simulink model "tx2"  (R2022a)
settings: Solver=FixedStepDiscrete  StartTime=0.0  StopTime=3.1e6  FixedStep=1  RelTol=1e-3
undefined symbols (not defined in the file or in its folder): rom_bf1, rom_bf2, rom_bf3, rom_bf4, rom_bf5, rom_bf6, rom_bf7, rom_bf8, rom_pilot_tt
libraries: hdlsllib x809, whdlutilities x460, whdlmod x104, whdledac x26, simulink x3
(part 3 of 27)

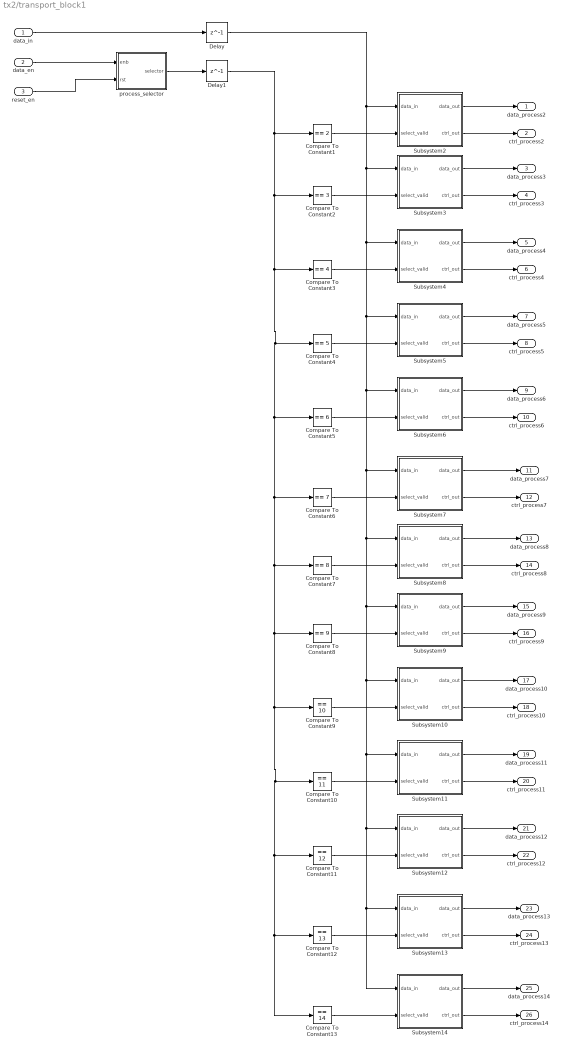
== system tx2/transport_block1 ==
  data_in : Inport  OutDataTypeStr=boolean
  data_en : Inport  Port=2  OutDataTypeStr=boolean
  reset_en : Inport  Port=3  OutDataTypeStr=boolean
  Compare To Constant1 : hdlsllib/Logic and Bit Operations/Compare To Constant  relop===  const=2  OutDataTypeStr=boolean
      settings: SourceProductBaseCode=SL
  Compare To Constant10 : hdlsllib/Logic and Bit Operations/Compare To Constant  relop===  const=11  OutDataTypeStr=boolean
      settings: SourceProductBaseCode=SL
  Compare To Constant11 : hdlsllib/Logic and Bit Operations/Compare To Constant  relop===  const=12  OutDataTypeStr=boolean
      settings: SourceProductBaseCode=SL
  Compare To Constant12 : hdlsllib/Logic and Bit Operations/Compare To Constant  relop===  const=13  OutDataTypeStr=boolean
      settings: SourceProductBaseCode=SL
  Compare To Constant13 : hdlsllib/Logic and Bit Operations/Compare To Constant  relop===  const=14  OutDataTypeStr=boolean
      settings: SourceProductBaseCode=SL
  Compare To Constant2 : hdlsllib/Logic and Bit Operations/Compare To Constant  relop===  const=3  OutDataTypeStr=boolean
      settings: SourceProductBaseCode=SL
  Compare To Constant3 : hdlsllib/Logic and Bit Operations/Compare To Constant  relop===  const=4  OutDataTypeStr=boolean
      settings: SourceProductBaseCode=SL
  Compare To Constant4 : hdlsllib/Logic and Bit Operations/Compare To Constant  relop===  const=5  OutDataTypeStr=boolean
      settings: SourceProductBaseCode=SL
  Compare To Constant5 : hdlsllib/Logic and Bit Operations/Compare To Constant  relop===  const=6  OutDataTypeStr=boolean
      settings: SourceProductBaseCode=SL
  Compare To Constant6 : hdlsllib/Logic and Bit Operations/Compare To Constant  relop===  const=7  OutDataTypeStr=boolean
      settings: SourceProductBaseCode=SL
  Compare To Constant7 : hdlsllib/Logic and Bit Operations/Compare To Constant  relop===  const=8  OutDataTypeStr=boolean
      settings: SourceProductBaseCode=SL
  Compare To Constant8 : hdlsllib/Logic and Bit Operations/Compare To Constant  relop===  const=9  OutDataTypeStr=boolean
      settings: SourceProductBaseCode=SL
  Compare To Constant9 : hdlsllib/Logic and Bit Operations/Compare To Constant  relop===  const=10  OutDataTypeStr=boolean
      settings: SourceProductBaseCode=SL
  Delay : Delay  DelayLength=1  InitialCondition=0
  Delay1 : Delay  DelayLength=1  InitialCondition=0
  Subsystem10 : Subsystem
  Subsystem11 : Subsystem
  Subsystem12 : Subsystem
  Subsystem13 : Subsystem
  Subsystem14 : Subsystem
  Subsystem2 : Subsystem
  Subsystem3 : Subsystem
  Subsystem4 : Subsystem
  Subsystem5 : Subsystem
  Subsystem6 : Subsystem
  Subsystem7 : Subsystem
  Subsystem8 : Subsystem
  Subsystem9 : Subsystem
  process_selector : Subsystem  mask{transblock_len=512, process_len=14}
      mask prompts: transblock_len "the length of the transport block"; process_len "the number of process"
      mask DialogControl ParameterGroupVar Prompt: 参数
  data_process2 : Outport  OutDataTypeStr=boolean  VectorParamsAs1DForOutWhenUnconnected=off
  ctrl_process2 : Outport  Port=2  OutDataTypeStr=Bus: samplecontrol  VectorParamsAs1DForOutWhenUnconnected=off
  data_process3 : Outport  Port=3  OutDataTypeStr=boolean  VectorParamsAs1DForOutWhenUnconnected=off
  ctrl_process3 : Outport  Port=4  OutDataTypeStr=Bus: samplecontrol  VectorParamsAs1DForOutWhenUnconnected=off
  data_process4 : Outport  Port=5  OutDataTypeStr=boolean  VectorParamsAs1DForOutWhenUnconnected=off
  ctrl_process4 : Outport  Port=6  OutDataTypeStr=Bus: samplecontrol  VectorParamsAs1DForOutWhenUnconnected=off
  data_process5 : Outport  Port=7  OutDataTypeStr=boolean  VectorParamsAs1DForOutWhenUnconnected=off
  ctrl_process5 : Outport  Port=8  OutDataTypeStr=Bus: samplecontrol  VectorParamsAs1DForOutWhenUnconnected=off
  data_process6 : Outport  Port=9  OutDataTypeStr=boolean  VectorParamsAs1DForOutWhenUnconnected=off
  ctrl_process6 : Outport  Port=10  OutDataTypeStr=Bus: samplecontrol  VectorParamsAs1DForOutWhenUnconnected=off
  data_process7 : Outport  Port=11  OutDataTypeStr=boolean  VectorParamsAs1DForOutWhenUnconnected=off
  ctrl_process7 : Outport  Port=12  OutDataTypeStr=Bus: samplecontrol  VectorParamsAs1DForOutWhenUnconnected=off
  data_process8 : Outport  Port=13  OutDataTypeStr=boolean  VectorParamsAs1DForOutWhenUnconnected=off
  ctrl_process8 : Outport  Port=14  OutDataTypeStr=Bus: samplecontrol  VectorParamsAs1DForOutWhenUnconnected=off
  data_process9 : Outport  Port=15  OutDataTypeStr=boolean  VectorParamsAs1DForOutWhenUnconnected=off
  ctrl_process9 : Outport  Port=16  OutDataTypeStr=Bus: samplecontrol  VectorParamsAs1DForOutWhenUnconnected=off
  data_process10 : Outport  Port=17  OutDataTypeStr=boolean  VectorParamsAs1DForOutWhenUnconnected=off
  ctrl_process10 : Outport  Port=18  OutDataTypeStr=Bus: samplecontrol  VectorParamsAs1DForOutWhenUnconnected=off
  data_process11 : Outport  Port=19  OutDataTypeStr=boolean  VectorParamsAs1DForOutWhenUnconnected=off
  ctrl_process11 : Outport  Port=20  OutDataTypeStr=Bus: samplecontrol  VectorParamsAs1DForOutWhenUnconnected=off
  data_process12 : Outport  Port=21  OutDataTypeStr=boolean  VectorParamsAs1DForOutWhenUnconnected=off
  ctrl_process12 : Outport  Port=22  OutDataTypeStr=Bus: samplecontrol  VectorParamsAs1DForOutWhenUnconnected=off
  data_process13 : Outport  Port=23  OutDataTypeStr=boolean  VectorParamsAs1DForOutWhenUnconnected=off
  ctrl_process13 : Outport  Port=24  OutDataTypeStr=Bus: samplecontrol  VectorParamsAs1DForOutWhenUnconnected=off
  data_process14 : Outport  Port=25  OutDataTypeStr=boolean  VectorParamsAs1DForOutWhenUnconnected=off
  ctrl_process14 : Outport  Port=26  OutDataTypeStr=Bus: samplecontrol  VectorParamsAs1DForOutWhenUnconnected=off
  wires:
  data_in/1 -> Delay/1
  data_en/1 -> process_selector/1(enb)
  process_selector/1(selector) -> Delay1/1
  Compare To Constant1/1 -> Subsystem2/2(select_valid)
  Subsystem2/1(data_out) -> data_process2/1
  Subsystem2/2(ctrl_out) -> ctrl_process2/1
  Compare To Constant2/1 -> Subsystem3/2(select_valid)
  Subsystem3/1(data_out) -> data_process3/1
  Subsystem3/2(ctrl_out) -> ctrl_process3/1
  Compare To Constant3/1 -> Subsystem4/2(select_valid)
  Subsystem4/1(data_out) -> data_process4/1
  Subsystem4/2(ctrl_out) -> ctrl_process4/1
  Compare To Constant4/1 -> Subsystem5/2(select_valid)
  Subsystem5/1(data_out) -> data_process5/1
  Subsystem5/2(ctrl_out) -> ctrl_process5/1
  Compare To Constant5/1 -> Subsystem6/2(select_valid)
  Subsystem6/1(data_out) -> data_process6/1
  Subsystem6/2(ctrl_out) -> ctrl_process6/1
  Compare To Constant6/1 -> Subsystem7/2(select_valid)
  Subsystem7/1(data_out) -> data_process7/1
  Subsystem7/2(ctrl_out) -> ctrl_process7/1
  Compare To Constant7/1 -> Subsystem8/2(select_valid)
  Subsystem8/1(data_out) -> data_process8/1
  Subsystem8/2(ctrl_out) -> ctrl_process8/1
  Subsystem13/2(ctrl_out) -> ctrl_process13/1
  Subsystem13/1(data_out) -> data_process13/1
  Compare To Constant12/1 -> Subsystem13/2(select_valid)
  Subsystem12/2(ctrl_out) -> ctrl_process12/1
  Subsystem12/1(data_out) -> data_process12/1
  Compare To Constant11/1 -> Subsystem12/2(select_valid)
  Subsystem11/2(ctrl_out) -> ctrl_process11/1
  Subsystem11/1(data_out) -> data_process11/1
  Compare To Constant10/1 -> Subsystem11/2(select_valid)
  Subsystem10/2(ctrl_out) -> ctrl_process10/1
  Subsystem10/1(data_out) -> data_process10/1
  Compare To Constant9/1 -> Subsystem10/2(select_valid)
  Subsystem9/2(ctrl_out) -> ctrl_process9/1
  Subsystem9/1(data_out) -> data_process9/1
  Compare To Constant8/1 -> Subsystem9/2(select_valid)
  reset_en/1 -> process_selector/2(rst)
  Delay1/1 -> Compare To Constant13/1, Compare To Constant12/1, Compare To Constant11/1, Compare To Constant10/1, Compare To Constant9/1, Compare To Constant8/1, Compare To Constant7/1, Compare To Constant6/1, Compare To Constant5/1, Compare To Constant4/1, Compare To Constant3/1, Compare To Constant2/1, Compare To Constant1/1
  Delay/1 -> Subsystem10/1(data_in), Subsystem12/1(data_in), Subsystem14/1(data_in), Subsystem13/1(data_in), Subsystem11/1(data_in), Subsystem9/1(data_in), Subsystem8/1(data_in), Subsystem7/1(data_in), Subsystem6/1(data_in), Subsystem5/1(data_in), Subsystem4/1(data_in), Subsystem3/1(data_in), Subsystem2/1(data_in)
  Compare To Constant13/1 -> Subsystem14/2(select_valid)
  Subsystem14/1(data_out) -> data_process14/1
  Subsystem14/2(ctrl_out) -> ctrl_process14/1

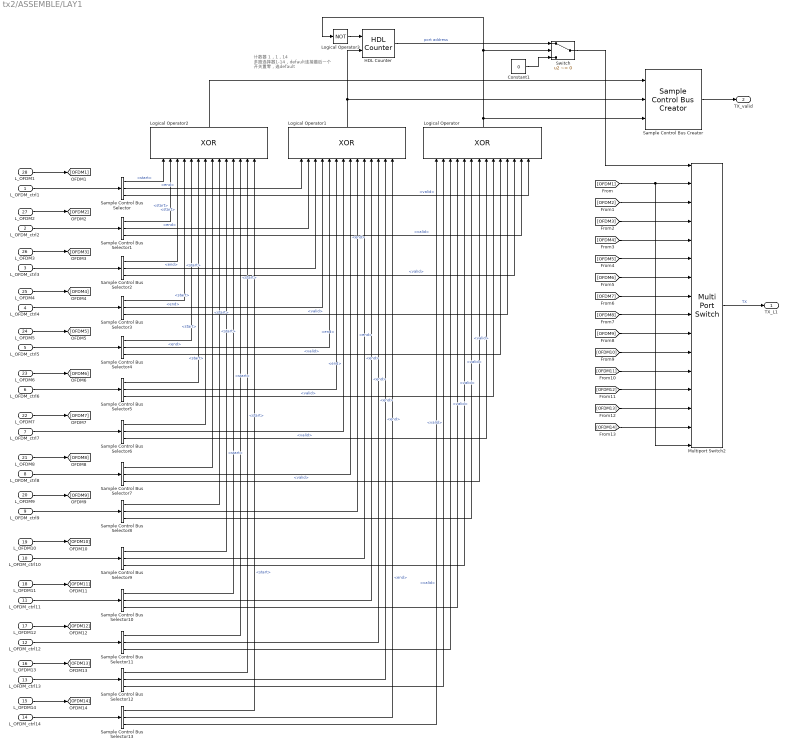
== system tx2/ASSEMBLE/LAY1 ==
  note: 计数器 1，1，14
      | 多路选择器1-14，default连接最后一个
      | 开关置零，选default
  L_OFDM_ctrl1 : Inport  OutDataTypeStr=Bus: samplecontrol
  L_OFDM_ctrl2 : Inport  Port=2  OutDataTypeStr=Bus: samplecontrol
  L_OFDM_ctrl3 : Inport  Port=3  OutDataTypeStr=Bus: samplecontrol
  L_OFDM_ctrl4 : Inport  Port=4  OutDataTypeStr=Bus: samplecontrol
  L_OFDM_ctrl5 : Inport  Port=5  OutDataTypeStr=Bus: samplecontrol
  L_OFDM_ctrl6 : Inport  Port=6  OutDataTypeStr=Bus: samplecontrol
  L_OFDM_ctrl7 : Inport  Port=7  OutDataTypeStr=Bus: samplecontrol
  L_OFDM_ctrl8 : Inport  Port=8  OutDataTypeStr=Bus: samplecontrol
  L_OFDM_ctrl9 : Inport  Port=9  OutDataTypeStr=Bus: samplecontrol
  L_OFDM_ctrl10 : Inport  Port=10  OutDataTypeStr=Bus: samplecontrol
  L_OFDM_ctrl11 : Inport  Port=11  OutDataTypeStr=Bus: samplecontrol
  L_OFDM_ctrl12 : Inport  Port=12  OutDataTypeStr=Bus: samplecontrol
  L_OFDM_ctrl13 : Inport  Port=13  OutDataTypeStr=Bus: samplecontrol
  L_OFDM_ctrl14 : Inport  Port=14  OutDataTypeStr=Bus: samplecontrol
  L_OFDM14 : Inport  Port=15
  L_OFDM13 : Inport  Port=16
  L_OFDM12 : Inport  Port=17
  L_OFDM11 : Inport  Port=18
  L_OFDM10 : Inport  Port=19
  L_OFDM9 : Inport  Port=20
  L_OFDM8 : Inport  Port=21
  L_OFDM7 : Inport  Port=22
  L_OFDM6 : Inport  Port=23
  L_OFDM5 : Inport  Port=24
  L_OFDM4 : Inport  Port=25
  L_OFDM3 : Inport  Port=26
  L_OFDM2 : Inport  Port=27
  L_OFDM1 : Inport  Port=28
  Constant1 : Constant  Value=0  OutDataTypeStr=uint8
  HDL Counter : hdlsllib/Sources/HDL Counter  CountType=Count limited  CountInit=0  CountStep=1  CountMax=13  CountFromType=Initial value  CountFrom=0  CountResetPort=on  CountLoadPort=off  CountEnbPort=on  CountDirPort=off  CountHitOutputPort=off  CountDataType=Unsigned  CountWordLen=8  CountFracLen=0  CountSampTime=1
  Logical Operator : Logic  Operator=XOR  Inputs=14  AllPortsSameDT=off  OutDataTypeStr=boolean
  Logical Operator1 : Logic  Operator=XOR  Inputs=14  AllPortsSameDT=off  OutDataTypeStr=boolean
  Logical Operator2 : Logic  Operator=XOR  Inputs=14  AllPortsSameDT=off  OutDataTypeStr=boolean
  Logical Operator3 : Logic  Operator=NOT  AllPortsSameDT=off  OutDataTypeStr=boolean
  Multiport Switch2 : MultiPortSwitch  DataPortOrder=Zero-based contiguous  Inputs=14  DataPortForDefault=Additional data port  zeroidx=on  SaturateOnIntegerOverflow=off  InputSameDT=off
  Sample Control Bus Creator : whdlutilities/Sample Control Bus Creator
      settings: SourceProductBaseCode=LH
  Sample Control Bus Selector{,1..13} (14 alike) : whdlutilities/Sample Control Bus Selector  OutputSignals=start,end,valid
      settings: SourceProductBaseCode=LH
  Switch : Switch  Criteria=u2 ~= 0  SaturateOnIntegerOverflow=off  InputSameDT=off
  TX_L1 : Outport
  TX_valid : Outport  Port=2  OutDataTypeStr=Bus: samplecontrol
  wires:
  Sample Control Bus Selector8/3 -> Logical Operator/6  "<valid>"
  L_OFDM_ctrl8/1 -> Sample Control Bus Selector7/1
  Sample Control Bus Selector10/3 -> Logical Operator/4  "<valid>"
  L_OFDM5/1 -> [OFDM5]
  Sample Control Bus Selector/3 -> Logical Operator/14  "<valid>"
  Sample Control Bus Selector10/2 -> Logical Operator1/11  "<end>"
  L_OFDM8/1 -> [OFDM8]
  Sample Control Bus Selector1/3 -> Logical Operator/13  "<valid>"
  L_OFDM3/1 -> [OFDM3]
  Sample Control Bus Selector12/3 -> Logical Operator/2  "<valid>"
  L_OFDM2/1 -> [OFDM2]
  Sample Control Bus Selector5/2 -> Logical Operator1/6  "<end>"
  Sample Control Bus Selector6/3 -> Logical Operator/8  "<valid>"
  Logical Operator/1 -> Logical Operator3/1, Switch/2, Sample Control Bus Creator/3
  Sample Control Bus Selector6/2 -> Logical Operator1/7  "<end>"
  L_OFDM10/1 -> [OFDM10]
  Sample Control Bus Selector13/2 -> Logical Operator1/14  "<end>"
  Sample Control Bus Selector12/2 -> Logical Operator1/13  "<end>"
  L_OFDM_ctrl6/1 -> Sample Control Bus Selector5/1
  L_OFDM_ctrl10/1 -> Sample Control Bus Selector9/1
  Sample Control Bus Selector7/3 -> Logical Operator/7  "<valid>"
  Sample Control Bus Selector8/2 -> Logical Operator1/9  "<end>"
  L_OFDM13/1 -> [OFDM13]
  HDL Counter/1 -> Switch/1  "port address"
  Sample Control Bus Selector2/3 -> Logical Operator/12  "<valid>"
  Switch/1 -> Multiport Switch2/1
  Sample Control Bus Selector5/3 -> Logical Operator/9  "<valid>"
  Sample Control Bus Selector/2 -> Logical Operator1/1  "<end>"
  L_OFDM12/1 -> [OFDM12]
  L_OFDM11/1 -> [OFDM11]
  Constant1/1 -> Switch/3
  L_OFDM1/1 -> [OFDM1]
  Sample Control Bus Selector2/2 -> Logical Operator1/3  "<end>"
  Sample Control Bus Selector4/3 -> Logical Operator/10  "<valid>"
  Sample Control Bus Selector11/2 -> Logical Operator1/12  "<end>"
  L_OFDM4/1 -> [OFDM4]
  Sample Control Bus Selector11/3 -> Logical Operator/3  "<valid>"
  Sample Control Bus Selector4/2 -> Logical Operator1/5  "<end>"
  Sample Control Bus Selector3/3 -> Logical Operator/11  "<valid>"
  Sample Control Bus Selector13/3 -> Logical Operator/1  "<valid>"
  Sample Control Bus Selector3/2 -> Logical Operator1/4  "<end>"
  Sample Control Bus Selector1/2 -> Logical Operator1/2  "<end>"
  L_OFDM_ctrl12/1 -> Sample Control Bus Selector11/1
  Sample Control Bus Selector7/2 -> Logical Operator1/8  "<end>"
  L_OFDM_ctrl5/1 -> Sample Control Bus Selector4/1
  Sample Control Bus Selector9/2 -> Logical Operator1/10  "<end>"
  Sample Control Bus Selector9/3 -> Logical Operator/5  "<valid>"
  L_OFDM_ctrl13/1 -> Sample Control Bus Selector12/1
  L_OFDM_ctrl2/1 -> Sample Control Bus Selector1/1
  L_OFDM14/1 -> [OFDM14]
  L_OFDM6/1 -> [OFDM6]
  L_OFDM7/1 -> [OFDM7]
  L_OFDM_ctrl3/1 -> Sample Control Bus Selector2/1
  L_OFDM_ctrl9/1 -> Sample Control Bus Selector8/1
  L_OFDM_ctrl14/1 -> Sample Control Bus Selector13/1
  L_OFDM_ctrl4/1 -> Sample Control Bus Selector3/1
  L_OFDM_ctrl7/1 -> Sample Control Bus Selector6/1
  L_OFDM_ctrl1/1 -> Sample Control Bus Selector/1
  L_OFDM9/1 -> [OFDM9]
  L_OFDM_ctrl11/1 -> Sample Control Bus Selector10/1
  Sample Control Bus Selector/1 -> Logical Operator2/1  "<start>"
  Sample Control Bus Selector1/1 -> Logical Operator2/2  "<start>"
  Sample Control Bus Selector2/1 -> Logical Operator2/3  "<start>"
  Sample Control Bus Selector3/1 -> Logical Operator2/4  "<start>"
  Sample Control Bus Selector4/1 -> Logical Operator2/5  "<start>"
  Sample Control Bus Selector5/1 -> Logical Operator2/6  "<start>"
  Sample Control Bus Selector6/1 -> Logical Operator2/7  "<start>"
  Sample Control Bus Selector7/1 -> Logical Operator2/8  "<start>"
  Sample Control Bus Selector8/1 -> Logical Operator2/9  "<start>"
  Sample Control Bus Selector9/1 -> Logical Operator2/10  "<start>"
  Sample Control Bus Selector10/1 -> Logical Operator2/11  "<start>"
  Sample Control Bus Selector11/1 -> Logical Operator2/12  "<start>"
  Sample Control Bus Selector12/1 -> Logical Operator2/13  "<start>"
  Sample Control Bus Selector13/1 -> Logical Operator2/14  "<start>"
  Sample Control Bus Creator/1 -> TX_valid/1
  Logical Operator2/1 -> Sample Control Bus Creator/1
  [OFDM2] -> Multiport Switch2/3
  [OFDM3] -> Multiport Switch2/4
  Multiport Switch2/1 -> TX_L1/1  "TX"
  Logical Operator3/1 -> HDL Counter/1
  Logical Operator1/1 -> HDL Counter/2, Sample Control Bus Creator/2
  [OFDM4] -> Multiport Switch2/5
  [OFDM5] -> Multiport Switch2/6
  [OFDM6] -> Multiport Switch2/7
  [OFDM7] -> Multiport Switch2/8
  [OFDM8] -> Multiport Switch2/9
  [OFDM9] -> Multiport Switch2/10
  [OFDM10] -> Multiport Switch2/11
  [OFDM11] -> Multiport Switch2/12
  [OFDM12] -> Multiport Switch2/13
  [OFDM13] -> Multiport Switch2/14
  [OFDM14] -> Multiport Switch2/15
  [OFDM1] -> Multiport Switch2/16, Multiport Switch2/2

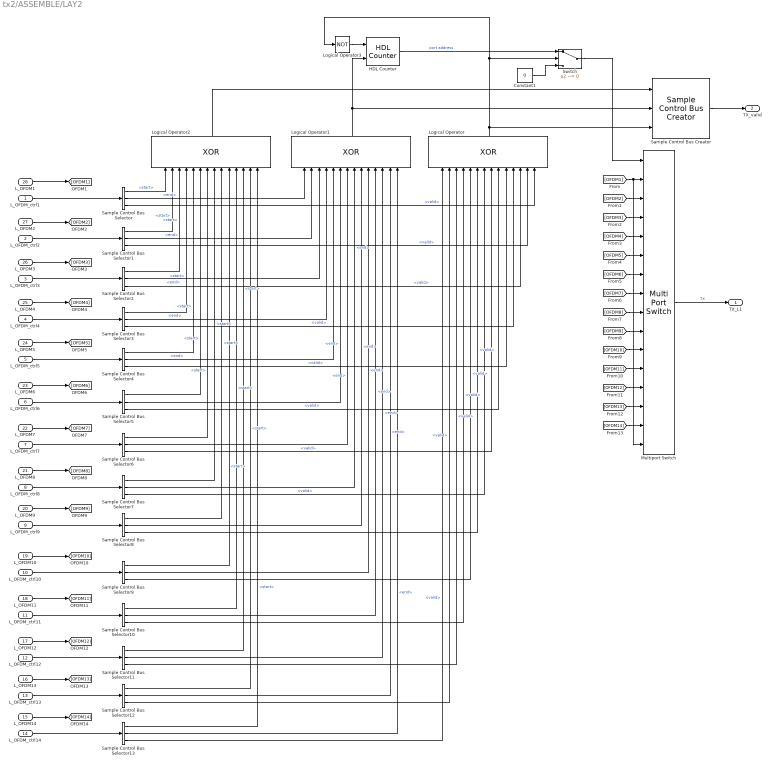
== system tx2/ASSEMBLE/LAY2 ==
  L_OFDM_ctrl1 : Inport  OutDataTypeStr=Bus: samplecontrol
  L_OFDM_ctrl2 : Inport  Port=2  OutDataTypeStr=Bus: samplecontrol
  L_OFDM_ctrl3 : Inport  Port=3  OutDataTypeStr=Bus: samplecontrol
  L_OFDM_ctrl4 : Inport  Port=4  OutDataTypeStr=Bus: samplecontrol
  L_OFDM_ctrl5 : Inport  Port=5  OutDataTypeStr=Bus: samplecontrol
  L_OFDM_ctrl6 : Inport  Port=6  OutDataTypeStr=Bus: samplecontrol
  L_OFDM_ctrl7 : Inport  Port=7  OutDataTypeStr=Bus: samplecontrol
  L_OFDM_ctrl8 : Inport  Port=8  OutDataTypeStr=Bus: samplecontrol
  L_OFDM_ctrl9 : Inport  Port=9  OutDataTypeStr=Bus: samplecontrol
  L_OFDM_ctrl10 : Inport  Port=10  OutDataTypeStr=Bus: samplecontrol
  L_OFDM_ctrl11 : Inport  Port=11  OutDataTypeStr=Bus: samplecontrol
  L_OFDM_ctrl12 : Inport  Port=12  OutDataTypeStr=Bus: samplecontrol
  L_OFDM_ctrl13 : Inport  Port=13  OutDataTypeStr=Bus: samplecontrol
  L_OFDM_ctrl14 : Inport  Port=14  OutDataTypeStr=Bus: samplecontrol
  L_OFDM14 : Inport  Port=15
  L_OFDM13 : Inport  Port=16
  L_OFDM12 : Inport  Port=17
  L_OFDM11 : Inport  Port=18
  L_OFDM10 : Inport  Port=19
  L_OFDM9 : Inport  Port=20
  L_OFDM8 : Inport  Port=21
  L_OFDM7 : Inport  Port=22
  L_OFDM6 : Inport  Port=23
  L_OFDM5 : Inport  Port=24
  L_OFDM4 : Inport  Port=25
  L_OFDM3 : Inport  Port=26
  L_OFDM2 : Inport  Port=27
  L_OFDM1 : Inport  Port=28
  Constant1 : Constant  Value=0  OutDataTypeStr=uint8
  HDL Counter : hdlsllib/Sources/HDL Counter  CountType=Count limited  CountInit=0  CountStep=1  CountMax=13  CountFromType=Initial value  CountFrom=0  CountResetPort=on  CountLoadPort=off  CountEnbPort=on  CountDirPort=off  CountHitOutputPort=off  CountDataType=Unsigned  CountWordLen=8  CountFracLen=0  CountSampTime=1
  Logical Operator : Logic  Operator=XOR  Inputs=14  AllPortsSameDT=off  OutDataTypeStr=boolean
  Logical Operator1 : Logic  Operator=XOR  Inputs=14  AllPortsSameDT=off  OutDataTypeStr=boolean
  Logical Operator2 : Logic  Operator=XOR  Inputs=14  AllPortsSameDT=off  OutDataTypeStr=boolean
  Logical Operator3 : Logic  Operator=NOT  AllPortsSameDT=off  OutDataTypeStr=boolean
  Multiport Switch : MultiPortSwitch  DataPortOrder=Zero-based contiguous  Inputs=14  DataPortForDefault=Additional data port  zeroidx=on  SaturateOnIntegerOverflow=off  InputSameDT=off
  Sample Control Bus Creator : whdlutilities/Sample Control Bus Creator
      settings: SourceProductBaseCode=LH
  Sample Control Bus Selector{,1..13} (14 alike) : whdlutilities/Sample Control Bus Selector  OutputSignals=start,end,valid
      settings: SourceProductBaseCode=LH
  Switch : Switch  Criteria=u2 ~= 0  SaturateOnIntegerOverflow=off  InputSameDT=off
  TX_L1 : Outport
  TX_valid : Outport  Port=2  OutDataTypeStr=Bus: samplecontrol
  wires:
  Logical Operator2/1 -> Sample Control Bus Creator/1
  Sample Control Bus Creator/1 -> TX_valid/1
  Sample Control Bus Selector13/1 -> Logical Operator2/14  "<start>"
  Sample Control Bus Selector12/1 -> Logical Operator2/13  "<start>"
  Sample Control Bus Selector11/1 -> Logical Operator2/12  "<start>"
  Sample Control Bus Selector10/1 -> Logical Operator2/11  "<start>"
  Sample Control Bus Selector9/1 -> Logical Operator2/10  "<start>"
  Sample Control Bus Selector8/1 -> Logical Operator2/9  "<start>"
  Sample Control Bus Selector7/1 -> Logical Operator2/8  "<start>"
  Sample Control Bus Selector6/1 -> Logical Operator2/7  "<start>"
  Sample Control Bus Selector5/1 -> Logical Operator2/6  "<start>"
  Sample Control Bus Selector4/1 -> Logical Operator2/5  "<start>"
  Sample Control Bus Selector3/1 -> Logical Operator2/4  "<start>"
  Sample Control Bus Selector2/1 -> Logical Operator2/3  "<start>"
  Sample Control Bus Selector1/1 -> Logical Operator2/2  "<start>"
  Sample Control Bus Selector/1 -> Logical Operator2/1  "<start>"
  Multiport Switch/1 -> TX_L1/1  "TX"
  L_OFDM_ctrl11/1 -> Sample Control Bus Selector10/1
  L_OFDM9/1 -> [OFDM9]
  L_OFDM_ctrl1/1 -> Sample Control Bus Selector/1
  L_OFDM_ctrl7/1 -> Sample Control Bus Selector6/1
  L_OFDM_ctrl4/1 -> Sample Control Bus Selector3/1
  L_OFDM_ctrl14/1 -> Sample Control Bus Selector13/1
  L_OFDM_ctrl9/1 -> Sample Control Bus Selector8/1
  L_OFDM_ctrl3/1 -> Sample Control Bus Selector2/1
  L_OFDM7/1 -> [OFDM7]
  L_OFDM6/1 -> [OFDM6]
  L_OFDM14/1 -> [OFDM14]
  L_OFDM_ctrl2/1 -> Sample Control Bus Selector1/1
  L_OFDM_ctrl13/1 -> Sample Control Bus Selector12/1
  Sample Control Bus Selector9/3 -> Logical Operator/5  "<valid>"
  Sample Control Bus Selector9/2 -> Logical Operator1/10  "<end>"
  L_OFDM_ctrl5/1 -> Sample Control Bus Selector4/1
  Sample Control Bus Selector7/2 -> Logical Operator1/8  "<end>"
  L_OFDM_ctrl12/1 -> Sample Control Bus Selector11/1
  [OFDM8] -> Multiport Switch/9
  Sample Control Bus Selector1/2 -> Logical Operator1/2  "<end>"
  Sample Control Bus Selector3/2 -> Logical Operator1/4  "<end>"
  Sample Control Bus Selector13/3 -> Logical Operator/1  "<valid>"
  Sample Control Bus Selector3/3 -> Logical Operator/11  "<valid>"
  [OFDM3] -> Multiport Switch/4
  Sample Control Bus Selector4/2 -> Logical Operator1/5  "<end>"
  Sample Control Bus Selector11/3 -> Logical Operator/3  "<valid>"
  [OFDM11] -> Multiport Switch/12
  L_OFDM4/1 -> [OFDM4]
  Sample Control Bus Selector11/2 -> Logical Operator1/12  "<end>"
  Sample Control Bus Selector4/3 -> Logical Operator/10  "<valid>"
  [OFDM12] -> Multiport Switch/13
  Sample Control Bus Selector2/2 -> Logical Operator1/3  "<end>"
  L_OFDM1/1 -> [OFDM1]
  Constant1/1 -> Switch/3
  L_OFDM11/1 -> [OFDM11]
  L_OFDM12/1 -> [OFDM12]
  Sample Control Bus Selector/2 -> Logical Operator1/1  "<end>"
  Sample Control Bus Selector5/3 -> Logical Operator/9  "<valid>"
  Switch/1 -> Multiport Switch/1
  Sample Control Bus Selector2/3 -> Logical Operator/12  "<valid>"
  [OFDM13] -> Multiport Switch/14
  [OFDM4] -> Multiport Switch/5
  [OFDM5] -> Multiport Switch/6
  HDL Counter/1 -> Switch/1  "port address"
  L_OFDM13/1 -> [OFDM13]
  [OFDM10] -> Multiport Switch/11
  Sample Control Bus Selector8/2 -> Logical Operator1/9  "<end>"
  Sample Control Bus Selector7/3 -> Logical Operator/7  "<valid>"
  L_OFDM_ctrl10/1 -> Sample Control Bus Selector9/1
  L_OFDM_ctrl6/1 -> Sample Control Bus Selector5/1
  [OFDM1] -> Multiport Switch/16, Multiport Switch/2
  Sample Control Bus Selector12/2 -> Logical Operator1/13  "<end>"
  Sample Control Bus Selector13/2 -> Logical Operator1/14  "<end>"
  L_OFDM10/1 -> [OFDM10]
  Sample Control Bus Selector6/2 -> Logical Operator1/7  "<end>"
  [OFDM7] -> Multiport Switch/8
  [OFDM6] -> Multiport Switch/7
  Logical Operator/1 -> Sample Control Bus Creator/3, Switch/2, Logical Operator3/1
  Sample Control Bus Selector6/3 -> Logical Operator/8  "<valid>"
  Sample Control Bus Selector5/2 -> Logical Operator1/6  "<end>"
  [OFDM9] -> Multiport Switch/10
  [OFDM2] -> Multiport Switch/3
  L_OFDM2/1 -> [OFDM2]
  Sample Control Bus Selector12/3 -> Logical Operator/2  "<valid>"
  L_OFDM3/1 -> [OFDM3]
  Sample Control Bus Selector1/3 -> Logical Operator/13  "<valid>"
  L_OFDM8/1 -> [OFDM8]
  Sample Control Bus Selector10/2 -> Logical Operator1/11  "<end>"
  Sample Control Bus Selector/3 -> Logical Operator/14  "<valid>"
  L_OFDM5/1 -> [OFDM5]
  Logical Operator1/1 -> Sample Control Bus Creator/2, HDL Counter/2
  [OFDM14] -> Multiport Switch/15
  Sample Control Bus Selector10/3 -> Logical Operator/4  "<valid>"
  L_OFDM_ctrl8/1 -> Sample Control Bus Selector7/1
  Sample Control Bus Selector8/3 -> Logical Operator/6  "<valid>"
  Logical Operator3/1 -> HDL Counter/1

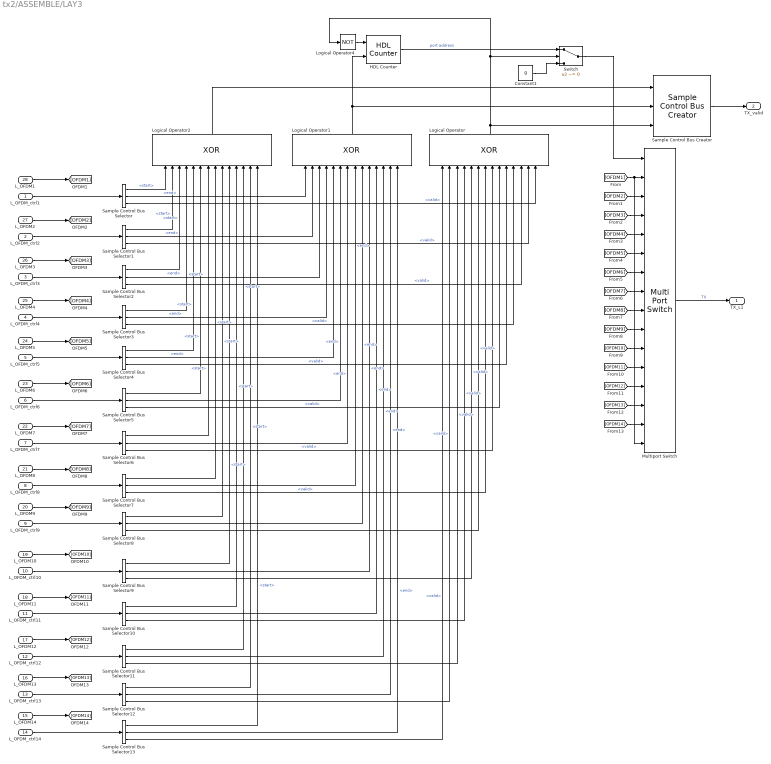
== system tx2/ASSEMBLE/LAY3 ==
  L_OFDM_ctrl1 : Inport  OutDataTypeStr=Bus: samplecontrol
  L_OFDM_ctrl2 : Inport  Port=2  OutDataTypeStr=Bus: samplecontrol
  L_OFDM_ctrl3 : Inport  Port=3  OutDataTypeStr=Bus: samplecontrol
  L_OFDM_ctrl4 : Inport  Port=4  OutDataTypeStr=Bus: samplecontrol
  L_OFDM_ctrl5 : Inport  Port=5  OutDataTypeStr=Bus: samplecontrol
  L_OFDM_ctrl6 : Inport  Port=6  OutDataTypeStr=Bus: samplecontrol
  L_OFDM_ctrl7 : Inport  Port=7  OutDataTypeStr=Bus: samplecontrol
  L_OFDM_ctrl8 : Inport  Port=8  OutDataTypeStr=Bus: samplecontrol
  L_OFDM_ctrl9 : Inport  Port=9  OutDataTypeStr=Bus: samplecontrol
  L_OFDM_ctrl10 : Inport  Port=10  OutDataTypeStr=Bus: samplecontrol
  L_OFDM_ctrl11 : Inport  Port=11  OutDataTypeStr=Bus: samplecontrol
  L_OFDM_ctrl12 : Inport  Port=12  OutDataTypeStr=Bus: samplecontrol
  L_OFDM_ctrl13 : Inport  Port=13  OutDataTypeStr=Bus: samplecontrol
  L_OFDM_ctrl14 : Inport  Port=14  OutDataTypeStr=Bus: samplecontrol
  L_OFDM14 : Inport  Port=15
  L_OFDM13 : Inport  Port=16
  L_OFDM12 : Inport  Port=17
  L_OFDM11 : Inport  Port=18
  L_OFDM10 : Inport  Port=19
  L_OFDM9 : Inport  Port=20
  L_OFDM8 : Inport  Port=21
  L_OFDM7 : Inport  Port=22
  L_OFDM6 : Inport  Port=23
  L_OFDM5 : Inport  Port=24
  L_OFDM4 : Inport  Port=25
  L_OFDM3 : Inport  Port=26
  L_OFDM2 : Inport  Port=27
  L_OFDM1 : Inport  Port=28
  Constant1 : Constant  Value=0  OutDataTypeStr=uint8
  HDL Counter : hdlsllib/Sources/HDL Counter  CountType=Count limited  CountInit=0  CountStep=1  CountMax=13  CountFromType=Initial value  CountFrom=0  CountResetPort=on  CountLoadPort=off  CountEnbPort=on  CountDirPort=off  CountHitOutputPort=off  CountDataType=Unsigned  CountWordLen=8  CountFracLen=0  CountSampTime=1
  Logical Operator : Logic  Operator=XOR  Inputs=14  AllPortsSameDT=off  OutDataTypeStr=boolean
  Logical Operator1 : Logic  Operator=XOR  Inputs=14  AllPortsSameDT=off  OutDataTypeStr=boolean
  Logical Operator2 : Logic  Operator=XOR  Inputs=14  AllPortsSameDT=off  OutDataTypeStr=boolean
  Logical Operator4 : Logic  Operator=NOT  AllPortsSameDT=off  OutDataTypeStr=boolean
  Multiport Switch : MultiPortSwitch  DataPortOrder=Zero-based contiguous  Inputs=14  DataPortForDefault=Additional data port  zeroidx=on  SaturateOnIntegerOverflow=off  InputSameDT=off
  Sample Control Bus Creator : whdlutilities/Sample Control Bus Creator
      settings: SourceProductBaseCode=LH
  Sample Control Bus Selector{,1..13} (14 alike) : whdlutilities/Sample Control Bus Selector  OutputSignals=start,end,valid
      settings: SourceProductBaseCode=LH
  Switch : Switch  Criteria=u2 ~= 0  SaturateOnIntegerOverflow=off  InputSameDT=off
  TX_L1 : Outport
  TX_valid : Outport  Port=2  OutDataTypeStr=Bus: samplecontrol
  wires:
  Sample Control Bus Selector8/3 -> Logical Operator/6  "<valid>"
  L_OFDM_ctrl8/1 -> Sample Control Bus Selector7/1
  Sample Control Bus Selector10/3 -> Logical Operator/4  "<valid>"
  [OFDM14] -> Multiport Switch/15
  Logical Operator1/1 -> HDL Counter/2, Sample Control Bus Creator/2
  L_OFDM5/1 -> [OFDM5]
  Sample Control Bus Selector/3 -> Logical Operator/14  "<valid>"
  Sample Control Bus Selector10/2 -> Logical Operator1/11  "<end>"
  L_OFDM8/1 -> [OFDM8]
  Sample Control Bus Selector1/3 -> Logical Operator/13  "<valid>"
  L_OFDM3/1 -> [OFDM3]
  Sample Control Bus Selector12/3 -> Logical Operator/2  "<valid>"
  L_OFDM2/1 -> [OFDM2]
  [OFDM2] -> Multiport Switch/3
  [OFDM9] -> Multiport Switch/10
  Sample Control Bus Selector5/2 -> Logical Operator1/6  "<end>"
  Sample Control Bus Selector6/3 -> Logical Operator/8  "<valid>"
  Logical Operator/1 -> Switch/2, Logical Operator4/1, Sample Control Bus Creator/3
  [OFDM6] -> Multiport Switch/7
  [OFDM7] -> Multiport Switch/8
  Sample Control Bus Selector6/2 -> Logical Operator1/7  "<end>"
  L_OFDM10/1 -> [OFDM10]
  Sample Control Bus Selector13/2 -> Logical Operator1/14  "<end>"
  Sample Control Bus Selector12/2 -> Logical Operator1/13  "<end>"
  [OFDM1] -> Multiport Switch/16, Multiport Switch/2
  L_OFDM_ctrl6/1 -> Sample Control Bus Selector5/1
  L_OFDM_ctrl10/1 -> Sample Control Bus Selector9/1
  Sample Control Bus Selector7/3 -> Logical Operator/7  "<valid>"
  Sample Control Bus Selector8/2 -> Logical Operator1/9  "<end>"
  [OFDM10] -> Multiport Switch/11
  L_OFDM13/1 -> [OFDM13]
  HDL Counter/1 -> Switch/1  "port address"
  [OFDM5] -> Multiport Switch/6
  [OFDM4] -> Multiport Switch/5
  [OFDM13] -> Multiport Switch/14
  Sample Control Bus Selector2/3 -> Logical Operator/12  "<valid>"
  Switch/1 -> Multiport Switch/1
  Sample Control Bus Selector5/3 -> Logical Operator/9  "<valid>"
  Sample Control Bus Selector/2 -> Logical Operator1/1  "<end>"
  L_OFDM12/1 -> [OFDM12]
  L_OFDM11/1 -> [OFDM11]
  Constant1/1 -> Switch/3
  L_OFDM1/1 -> [OFDM1]
  Sample Control Bus Selector2/2 -> Logical Operator1/3  "<end>"
  [OFDM12] -> Multiport Switch/13
  Sample Control Bus Selector4/3 -> Logical Operator/10  "<valid>"
  Sample Control Bus Selector11/2 -> Logical Operator1/12  "<end>"
  L_OFDM4/1 -> [OFDM4]
  [OFDM11] -> Multiport Switch/12
  Sample Control Bus Selector11/3 -> Logical Operator/3  "<valid>"
  Sample Control Bus Selector4/2 -> Logical Operator1/5  "<end>"
  [OFDM3] -> Multiport Switch/4
  Sample Control Bus Selector3/3 -> Logical Operator/11  "<valid>"
  Sample Control Bus Selector13/3 -> Logical Operator/1  "<valid>"
  Sample Control Bus Selector3/2 -> Logical Operator1/4  "<end>"
  Sample Control Bus Selector1/2 -> Logical Operator1/2  "<end>"
  [OFDM8] -> Multiport Switch/9
  L_OFDM_ctrl12/1 -> Sample Control Bus Selector11/1
  Sample Control Bus Selector7/2 -> Logical Operator1/8  "<end>"
  L_OFDM_ctrl5/1 -> Sample Control Bus Selector4/1
  Sample Control Bus Selector9/2 -> Logical Operator1/10  "<end>"
  Sample Control Bus Selector9/3 -> Logical Operator/5  "<valid>"
  L_OFDM_ctrl13/1 -> Sample Control Bus Selector12/1
  L_OFDM_ctrl2/1 -> Sample Control Bus Selector1/1
  L_OFDM14/1 -> [OFDM14]
  L_OFDM6/1 -> [OFDM6]
  L_OFDM7/1 -> [OFDM7]
  L_OFDM_ctrl3/1 -> Sample Control Bus Selector2/1
  L_OFDM_ctrl9/1 -> Sample Control Bus Selector8/1
  L_OFDM_ctrl14/1 -> Sample Control Bus Selector13/1
  L_OFDM_ctrl4/1 -> Sample Control Bus Selector3/1
  L_OFDM_ctrl7/1 -> Sample Control Bus Selector6/1
  L_OFDM_ctrl1/1 -> Sample Control Bus Selector/1
  L_OFDM9/1 -> [OFDM9]
  L_OFDM_ctrl11/1 -> Sample Control Bus Selector10/1
  Multiport Switch/1 -> TX_L1/1  "TX"
  Sample Control Bus Selector/1 -> Logical Operator2/1  "<start>"
  Sample Control Bus Selector1/1 -> Logical Operator2/2  "<start>"
  Sample Control Bus Selector2/1 -> Logical Operator2/3  "<start>"
  Sample Control Bus Selector3/1 -> Logical Operator2/4  "<start>"
  Sample Control Bus Selector4/1 -> Logical Operator2/5  "<start>"
  Sample Control Bus Selector5/1 -> Logical Operator2/6  "<start>"
  Sample Control Bus Selector6/1 -> Logical Operator2/7  "<start>"
  Sample Control Bus Selector7/1 -> Logical Operator2/8  "<start>"
  Sample Control Bus Selector8/1 -> Logical Operator2/9  "<start>"
  Sample Control Bus Selector9/1 -> Logical Operator2/10  "<start>"
  Sample Control Bus Selector10/1 -> Logical Operator2/11  "<start>"
  Sample Control Bus Selector11/1 -> Logical Operator2/12  "<start>"
  Sample Control Bus Selector12/1 -> Logical Operator2/13  "<start>"
  Sample Control Bus Selector13/1 -> Logical Operator2/14  "<start>"
  Sample Control Bus Creator/1 -> TX_valid/1
  Logical Operator2/1 -> Sample Control Bus Creator/1
  Logical Operator4/1 -> HDL Counter/1

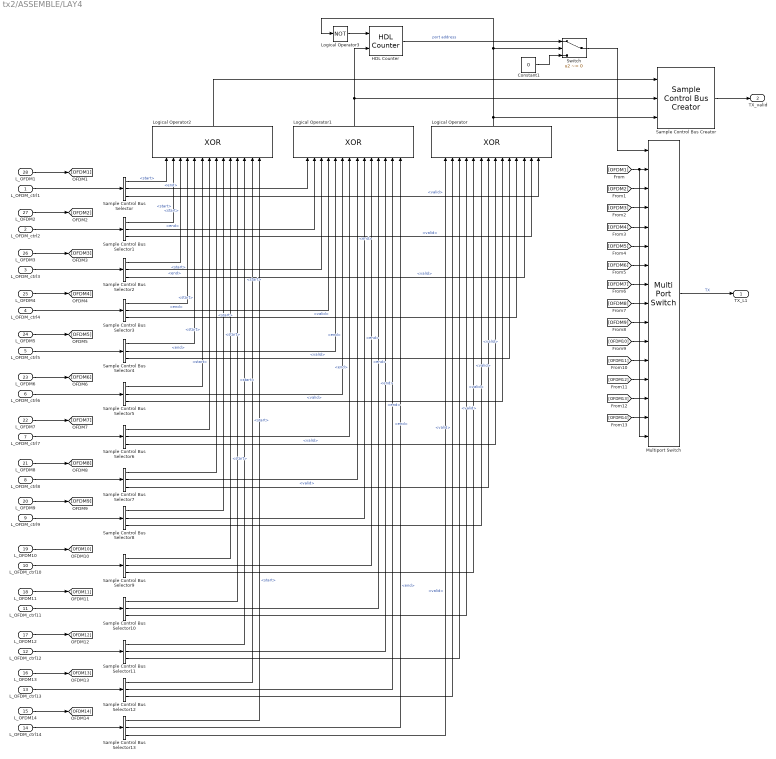
== system tx2/ASSEMBLE/LAY4 ==
  L_OFDM_ctrl1 : Inport  OutDataTypeStr=Bus: samplecontrol
  L_OFDM_ctrl2 : Inport  Port=2  OutDataTypeStr=Bus: samplecontrol
  L_OFDM_ctrl3 : Inport  Port=3  OutDataTypeStr=Bus: samplecontrol
  L_OFDM_ctrl4 : Inport  Port=4  OutDataTypeStr=Bus: samplecontrol
  L_OFDM_ctrl5 : Inport  Port=5  OutDataTypeStr=Bus: samplecontrol
  L_OFDM_ctrl6 : Inport  Port=6  OutDataTypeStr=Bus: samplecontrol
  L_OFDM_ctrl7 : Inport  Port=7  OutDataTypeStr=Bus: samplecontrol
  L_OFDM_ctrl8 : Inport  Port=8  OutDataTypeStr=Bus: samplecontrol
  L_OFDM_ctrl9 : Inport  Port=9  OutDataTypeStr=Bus: samplecontrol
  L_OFDM_ctrl10 : Inport  Port=10  OutDataTypeStr=Bus: samplecontrol
  L_OFDM_ctrl11 : Inport  Port=11  OutDataTypeStr=Bus: samplecontrol
  L_OFDM_ctrl12 : Inport  Port=12  OutDataTypeStr=Bus: samplecontrol
  L_OFDM_ctrl13 : Inport  Port=13  OutDataTypeStr=Bus: samplecontrol
  L_OFDM_ctrl14 : Inport  Port=14  OutDataTypeStr=Bus: samplecontrol
  L_OFDM14 : Inport  Port=15
  L_OFDM13 : Inport  Port=16
  L_OFDM12 : Inport  Port=17
  L_OFDM11 : Inport  Port=18
  L_OFDM10 : Inport  Port=19
  L_OFDM9 : Inport  Port=20
  L_OFDM8 : Inport  Port=21
  L_OFDM7 : Inport  Port=22
  L_OFDM6 : Inport  Port=23
  L_OFDM5 : Inport  Port=24
  L_OFDM4 : Inport  Port=25
  L_OFDM3 : Inport  Port=26
  L_OFDM2 : Inport  Port=27
  L_OFDM1 : Inport  Port=28
  Constant1 : Constant  Value=0  OutDataTypeStr=uint8
  HDL Counter : hdlsllib/Sources/HDL Counter  CountType=Count limited  CountInit=0  CountStep=1  CountMax=13  CountFromType=Initial value  CountFrom=0  CountResetPort=on  CountLoadPort=off  CountEnbPort=on  CountDirPort=off  CountHitOutputPort=off  CountDataType=Unsigned  CountWordLen=8  CountFracLen=0  CountSampTime=1
  Logical Operator : Logic  Operator=XOR  Inputs=14  AllPortsSameDT=off  OutDataTypeStr=boolean
  Logical Operator1 : Logic  Operator=XOR  Inputs=14  AllPortsSameDT=off  OutDataTypeStr=boolean
  Logical Operator2 : Logic  Operator=XOR  Inputs=14  AllPortsSameDT=off  OutDataTypeStr=boolean
  Logical Operator3 : Logic  Operator=NOT  AllPortsSameDT=off  OutDataTypeStr=boolean
  Multiport Switch : MultiPortSwitch  DataPortOrder=Zero-based contiguous  Inputs=14  DataPortForDefault=Additional data port  zeroidx=on  SaturateOnIntegerOverflow=off  InputSameDT=off
  Sample Control Bus Creator : whdlutilities/Sample Control Bus Creator
      settings: SourceProductBaseCode=LH
  Sample Control Bus Selector{,1..13} (14 alike) : whdlutilities/Sample Control Bus Selector  OutputSignals=start,end,valid
      settings: SourceProductBaseCode=LH
  Switch : Switch  Criteria=u2 ~= 0  SaturateOnIntegerOverflow=off  InputSameDT=off
  TX_L1 : Outport
  TX_valid : Outport  Port=2  OutDataTypeStr=Bus: samplecontrol
  wires:
  Logical Operator2/1 -> Sample Control Bus Creator/1
  Sample Control Bus Creator/1 -> TX_valid/1
  Sample Control Bus Selector13/1 -> Logical Operator2/14  "<start>"
  Sample Control Bus Selector12/1 -> Logical Operator2/13  "<start>"
  Sample Control Bus Selector11/1 -> Logical Operator2/12  "<start>"
  Sample Control Bus Selector10/1 -> Logical Operator2/11  "<start>"
  Sample Control Bus Selector9/1 -> Logical Operator2/10  "<start>"
  Sample Control Bus Selector8/1 -> Logical Operator2/9  "<start>"
  Sample Control Bus Selector7/1 -> Logical Operator2/8  "<start>"
  Sample Control Bus Selector6/1 -> Logical Operator2/7  "<start>"
  Sample Control Bus Selector5/1 -> Logical Operator2/6  "<start>"
  Sample Control Bus Selector4/1 -> Logical Operator2/5  "<start>"
  Sample Control Bus Selector3/1 -> Logical Operator2/4  "<start>"
  Sample Control Bus Selector2/1 -> Logical Operator2/3  "<start>"
  Sample Control Bus Selector1/1 -> Logical Operator2/2  "<start>"
  Sample Control Bus Selector/1 -> Logical Operator2/1  "<start>"
  Multiport Switch/1 -> TX_L1/1  "TX"
  L_OFDM_ctrl11/1 -> Sample Control Bus Selector10/1
  L_OFDM9/1 -> [OFDM9]
  L_OFDM_ctrl1/1 -> Sample Control Bus Selector/1
  L_OFDM_ctrl7/1 -> Sample Control Bus Selector6/1
  L_OFDM_ctrl4/1 -> Sample Control Bus Selector3/1
  L_OFDM_ctrl14/1 -> Sample Control Bus Selector13/1
  L_OFDM_ctrl9/1 -> Sample Control Bus Selector8/1
  L_OFDM_ctrl3/1 -> Sample Control Bus Selector2/1
  L_OFDM7/1 -> [OFDM7]
  L_OFDM6/1 -> [OFDM6]
  L_OFDM14/1 -> [OFDM14]
  L_OFDM_ctrl2/1 -> Sample Control Bus Selector1/1
  L_OFDM_ctrl13/1 -> Sample Control Bus Selector12/1
  Sample Control Bus Selector9/3 -> Logical Operator/5  "<valid>"
  Sample Control Bus Selector9/2 -> Logical Operator1/10  "<end>"
  L_OFDM_ctrl5/1 -> Sample Control Bus Selector4/1
  Sample Control Bus Selector7/2 -> Logical Operator1/8  "<end>"
  L_OFDM_ctrl12/1 -> Sample Control Bus Selector11/1
  [OFDM8] -> Multiport Switch/9
  Sample Control Bus Selector1/2 -> Logical Operator1/2  "<end>"
  Sample Control Bus Selector3/2 -> Logical Operator1/4  "<end>"
  Sample Control Bus Selector13/3 -> Logical Operator/1  "<valid>"
  Sample Control Bus Selector3/3 -> Logical Operator/11  "<valid>"
  [OFDM3] -> Multiport Switch/4
  Sample Control Bus Selector4/2 -> Logical Operator1/5  "<end>"
  Sample Control Bus Selector11/3 -> Logical Operator/3  "<valid>"
  [OFDM11] -> Multiport Switch/12
  L_OFDM4/1 -> [OFDM4]
  Sample Control Bus Selector11/2 -> Logical Operator1/12  "<end>"
  Sample Control Bus Selector4/3 -> Logical Operator/10  "<valid>"
  [OFDM12] -> Multiport Switch/13
  Sample Control Bus Selector2/2 -> Logical Operator1/3  "<end>"
  L_OFDM1/1 -> [OFDM1]
  Constant1/1 -> Switch/3
  L_OFDM11/1 -> [OFDM11]
  L_OFDM12/1 -> [OFDM12]
  Sample Control Bus Selector/2 -> Logical Operator1/1  "<end>"
  Sample Control Bus Selector5/3 -> Logical Operator/9  "<valid>"
  Switch/1 -> Multiport Switch/1
  Sample Control Bus Selector2/3 -> Logical Operator/12  "<valid>"
  [OFDM13] -> Multiport Switch/14
  [OFDM4] -> Multiport Switch/5
  [OFDM5] -> Multiport Switch/6
  HDL Counter/1 -> Switch/1  "port address"
  L_OFDM13/1 -> [OFDM13]
  [OFDM10] -> Multiport Switch/11
  Sample Control Bus Selector8/2 -> Logical Operator1/9  "<end>"
  Sample Control Bus Selector7/3 -> Logical Operator/7  "<valid>"
  L_OFDM_ctrl10/1 -> Sample Control Bus Selector9/1
  L_OFDM_ctrl6/1 -> Sample Control Bus Selector5/1
  Sample Control Bus Selector12/2 -> Logical Operator1/13  "<end>"
  Sample Control Bus Selector13/2 -> Logical Operator1/14  "<end>"
  L_OFDM10/1 -> [OFDM10]
  Sample Control Bus Selector6/2 -> Logical Operator1/7  "<end>"
  [OFDM7] -> Multiport Switch/8
  [OFDM6] -> Multiport Switch/7
  Logical Operator/1 -> Sample Control Bus Creator/3, Switch/2, Logical Operator3/1
  Sample Control Bus Selector6/3 -> Logical Operator/8  "<valid>"
  Sample Control Bus Selector5/2 -> Logical Operator1/6  "<end>"
  [OFDM9] -> Multiport Switch/10
  [OFDM2] -> Multiport Switch/3
  L_OFDM2/1 -> [OFDM2]
  Sample Control Bus Selector12/3 -> Logical Operator/2  "<valid>"
  L_OFDM3/1 -> [OFDM3]
  Sample Control Bus Selector1/3 -> Logical Operator/13  "<valid>"
  L_OFDM8/1 -> [OFDM8]
  Sample Control Bus Selector10/2 -> Logical Operator1/11  "<end>"
  Sample Control Bus Selector/3 -> Logical Operator/14  "<valid>"
  L_OFDM5/1 -> [OFDM5]
  Logical Operator1/1 -> Sample Control Bus Creator/2, HDL Counter/2
  [OFDM14] -> Multiport Switch/15
  Sample Control Bus Selector10/3 -> Logical Operator/4  "<valid>"
  L_OFDM_ctrl8/1 -> Sample Control Bus Selector7/1
  Sample Control Bus Selector8/3 -> Logical Operator/6  "<valid>"
  Logical Operator3/1 -> HDL Counter/1
  [OFDM1] -> Multiport Switch/16, Multiport Switch/2

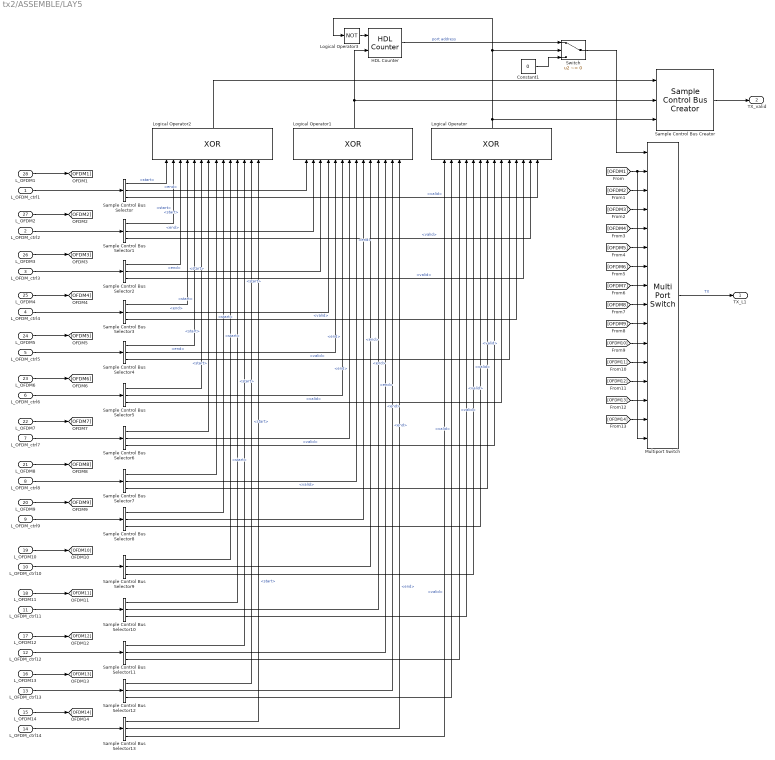
== system tx2/ASSEMBLE/LAY5 ==
  L_OFDM_ctrl1 : Inport  OutDataTypeStr=Bus: samplecontrol
  L_OFDM_ctrl2 : Inport  Port=2  OutDataTypeStr=Bus: samplecontrol
  L_OFDM_ctrl3 : Inport  Port=3  OutDataTypeStr=Bus: samplecontrol
  L_OFDM_ctrl4 : Inport  Port=4  OutDataTypeStr=Bus: samplecontrol
  L_OFDM_ctrl5 : Inport  Port=5  OutDataTypeStr=Bus: samplecontrol
  L_OFDM_ctrl6 : Inport  Port=6  OutDataTypeStr=Bus: samplecontrol
  L_OFDM_ctrl7 : Inport  Port=7  OutDataTypeStr=Bus: samplecontrol
  L_OFDM_ctrl8 : Inport  Port=8  OutDataTypeStr=Bus: samplecontrol
  L_OFDM_ctrl9 : Inport  Port=9  OutDataTypeStr=Bus: samplecontrol
  L_OFDM_ctrl10 : Inport  Port=10  OutDataTypeStr=Bus: samplecontrol
  L_OFDM_ctrl11 : Inport  Port=11  OutDataTypeStr=Bus: samplecontrol
  L_OFDM_ctrl12 : Inport  Port=12  OutDataTypeStr=Bus: samplecontrol
  L_OFDM_ctrl13 : Inport  Port=13  OutDataTypeStr=Bus: samplecontrol
  L_OFDM_ctrl14 : Inport  Port=14  OutDataTypeStr=Bus: samplecontrol
  L_OFDM14 : Inport  Port=15
  L_OFDM13 : Inport  Port=16
  L_OFDM12 : Inport  Port=17
  L_OFDM11 : Inport  Port=18
  L_OFDM10 : Inport  Port=19
  L_OFDM9 : Inport  Port=20
  L_OFDM8 : Inport  Port=21
  L_OFDM7 : Inport  Port=22
  L_OFDM6 : Inport  Port=23
  L_OFDM5 : Inport  Port=24
  L_OFDM4 : Inport  Port=25
  L_OFDM3 : Inport  Port=26
  L_OFDM2 : Inport  Port=27
  L_OFDM1 : Inport  Port=28
  Constant1 : Constant  Value=0  OutDataTypeStr=uint8
  HDL Counter : hdlsllib/Sources/HDL Counter  CountType=Count limited  CountInit=0  CountStep=1  CountMax=13  CountFromType=Initial value  CountFrom=0  CountResetPort=on  CountLoadPort=off  CountEnbPort=on  CountDirPort=off  CountHitOutputPort=off  CountDataType=Unsigned  CountWordLen=8  CountFracLen=0  CountSampTime=1
  Logical Operator : Logic  Operator=XOR  Inputs=14  AllPortsSameDT=off  OutDataTypeStr=boolean
  Logical Operator1 : Logic  Operator=XOR  Inputs=14  AllPortsSameDT=off  OutDataTypeStr=boolean
  Logical Operator2 : Logic  Operator=XOR  Inputs=14  AllPortsSameDT=off  OutDataTypeStr=boolean
  Logical Operator3 : Logic  Operator=NOT  AllPortsSameDT=off  OutDataTypeStr=boolean
  Multiport Switch : MultiPortSwitch  DataPortOrder=Zero-based contiguous  Inputs=14  DataPortForDefault=Additional data port  zeroidx=on  SaturateOnIntegerOverflow=off  InputSameDT=off
  Sample Control Bus Creator : whdlutilities/Sample Control Bus Creator
      settings: SourceProductBaseCode=LH
  Sample Control Bus Selector{,1..13} (14 alike) : whdlutilities/Sample Control Bus Selector  OutputSignals=start,end,valid
      settings: SourceProductBaseCode=LH
  Switch : Switch  Criteria=u2 ~= 0  SaturateOnIntegerOverflow=off  InputSameDT=off
  TX_L1 : Outport
  TX_valid : Outport  Port=2  OutDataTypeStr=Bus: samplecontrol
  wires:
  Sample Control Bus Selector8/3 -> Logical Operator/6  "<valid>"
  L_OFDM_ctrl8/1 -> Sample Control Bus Selector7/1
  Sample Control Bus Selector10/3 -> Logical Operator/4  "<valid>"
  [OFDM14] -> Multiport Switch/15
  Logical Operator1/1 -> HDL Counter/2, Sample Control Bus Creator/2
  L_OFDM5/1 -> [OFDM5]
  Sample Control Bus Selector/3 -> Logical Operator/14  "<valid>"
  Sample Control Bus Selector10/2 -> Logical Operator1/11  "<end>"
  L_OFDM8/1 -> [OFDM8]
  Sample Control Bus Selector1/3 -> Logical Operator/13  "<valid>"
  L_OFDM3/1 -> [OFDM3]
  Sample Control Bus Selector12/3 -> Logical Operator/2  "<valid>"
  L_OFDM2/1 -> [OFDM2]
  [OFDM2] -> Multiport Switch/3
  [OFDM9] -> Multiport Switch/10
  Sample Control Bus Selector5/2 -> Logical Operator1/6  "<end>"
  Sample Control Bus Selector6/3 -> Logical Operator/8  "<valid>"
  Logical Operator/1 -> Switch/2, Logical Operator3/1, Sample Control Bus Creator/3
  [OFDM6] -> Multiport Switch/7
  [OFDM7] -> Multiport Switch/8
  Sample Control Bus Selector6/2 -> Logical Operator1/7  "<end>"
  L_OFDM10/1 -> [OFDM10]
  Sample Control Bus Selector13/2 -> Logical Operator1/14  "<end>"
  Sample Control Bus Selector12/2 -> Logical Operator1/13  "<end>"
  [OFDM1] -> Multiport Switch/16, Multiport Switch/2
  L_OFDM_ctrl6/1 -> Sample Control Bus Selector5/1
  L_OFDM_ctrl10/1 -> Sample Control Bus Selector9/1
  Sample Control Bus Selector7/3 -> Logical Operator/7  "<valid>"
  Sample Control Bus Selector8/2 -> Logical Operator1/9  "<end>"
  [OFDM10] -> Multiport Switch/11
  L_OFDM13/1 -> [OFDM13]
  HDL Counter/1 -> Switch/1  "port address"
  [OFDM5] -> Multiport Switch/6
  [OFDM4] -> Multiport Switch/5
  [OFDM13] -> Multiport Switch/14
  Sample Control Bus Selector2/3 -> Logical Operator/12  "<valid>"
  Switch/1 -> Multiport Switch/1
  Sample Control Bus Selector5/3 -> Logical Operator/9  "<valid>"
  Sample Control Bus Selector/2 -> Logical Operator1/1  "<end>"
  L_OFDM12/1 -> [OFDM12]
  L_OFDM11/1 -> [OFDM11]
  Constant1/1 -> Switch/3
  L_OFDM1/1 -> [OFDM1]
  Sample Control Bus Selector2/2 -> Logical Operator1/3  "<end>"
  [OFDM12] -> Multiport Switch/13
  Sample Control Bus Selector4/3 -> Logical Operator/10  "<valid>"
  Sample Control Bus Selector11/2 -> Logical Operator1/12  "<end>"
  L_OFDM4/1 -> [OFDM4]
  [OFDM11] -> Multiport Switch/12
  Sample Control Bus Selector11/3 -> Logical Operator/3  "<valid>"
  Sample Control Bus Selector4/2 -> Logical Operator1/5  "<end>"
  [OFDM3] -> Multiport Switch/4
  Sample Control Bus Selector3/3 -> Logical Operator/11  "<valid>"
  Sample Control Bus Selector13/3 -> Logical Operator/1  "<valid>"
  Sample Control Bus Selector3/2 -> Logical Operator1/4  "<end>"
  Sample Control Bus Selector1/2 -> Logical Operator1/2  "<end>"
  [OFDM8] -> Multiport Switch/9
  L_OFDM_ctrl12/1 -> Sample Control Bus Selector11/1
  Sample Control Bus Selector7/2 -> Logical Operator1/8  "<end>"
  L_OFDM_ctrl5/1 -> Sample Control Bus Selector4/1
  Sample Control Bus Selector9/2 -> Logical Operator1/10  "<end>"
  Sample Control Bus Selector9/3 -> Logical Operator/5  "<valid>"
  L_OFDM_ctrl13/1 -> Sample Control Bus Selector12/1
  L_OFDM_ctrl2/1 -> Sample Control Bus Selector1/1
  L_OFDM14/1 -> [OFDM14]
  L_OFDM6/1 -> [OFDM6]
  L_OFDM7/1 -> [OFDM7]
  L_OFDM_ctrl3/1 -> Sample Control Bus Selector2/1
  L_OFDM_ctrl9/1 -> Sample Control Bus Selector8/1
  L_OFDM_ctrl14/1 -> Sample Control Bus Selector13/1
  L_OFDM_ctrl4/1 -> Sample Control Bus Selector3/1
  L_OFDM_ctrl7/1 -> Sample Control Bus Selector6/1
  L_OFDM_ctrl1/1 -> Sample Control Bus Selector/1
  L_OFDM9/1 -> [OFDM9]
  L_OFDM_ctrl11/1 -> Sample Control Bus Selector10/1
  Multiport Switch/1 -> TX_L1/1  "TX"
  Sample Control Bus Selector/1 -> Logical Operator2/1  "<start>"
  Sample Control Bus Selector1/1 -> Logical Operator2/2  "<start>"
  Sample Control Bus Selector2/1 -> Logical Operator2/3  "<start>"
  Sample Control Bus Selector3/1 -> Logical Operator2/4  "<start>"
  Sample Control Bus Selector4/1 -> Logical Operator2/5  "<start>"
  Sample Control Bus Selector5/1 -> Logical Operator2/6  "<start>"
  Sample Control Bus Selector6/1 -> Logical Operator2/7  "<start>"
  Sample Control Bus Selector7/1 -> Logical Operator2/8  "<start>"
  Sample Control Bus Selector8/1 -> Logical Operator2/9  "<start>"
  Sample Control Bus Selector9/1 -> Logical Operator2/10  "<start>"
  Sample Control Bus Selector10/1 -> Logical Operator2/11  "<start>"
  Sample Control Bus Selector11/1 -> Logical Operator2/12  "<start>"
  Sample Control Bus Selector12/1 -> Logical Operator2/13  "<start>"
  Sample Control Bus Selector13/1 -> Logical Operator2/14  "<start>"
  Sample Control Bus Creator/1 -> TX_valid/1
  Logical Operator2/1 -> Sample Control Bus Creator/1
  Logical Operator3/1 -> HDL Counter/1
